simulink model "ex3_2"  (Simulink 7.4)
settings: Solver=FixedStepDiscrete  SolverMode=SingleTasking  StartTime=0.0  StopTime=inf  FixedStep=0.005  RelTol=1e-3
libraries: dspsigops x20, dsparch4 x1
settings Model: Creator=fwornle  LastModifiedBy=fw  SimulationMode=external
settings ConfigSet: Description=rtmc9s12target_R2009b
settings DataIOCC: SignalLoggingName=sigsOut
settings OptimizationCC: InitFltsAndDblsToZero=on  OptimizeModelRefInitCode=on  LifeSpan=1
settings DebuggingCC: SaveWithParameterizedLinksMsg=none  SignalResolutionControl=TryResolveAllWithWarning  SolverPrmCheckMsg=none  MultiTaskDSMMsg=warning  MultiTaskCondExecSysMsg=none  StrictBusMsg=None
settings HardwareCC: ProdBitPerInt=16  ProdEndianess=BigEndian  ProdWordSize=16  ProdHWDeviceType=Motorola HC12
settings RTWCC: SystemTargetFile=mc9s12.tlc  GenerateMakefile=off  TemplateMakefile=mc9s12.tmf  ProcessScript=mc9s12_make_rtw_hook  IncludeERTFirstTime=on
settings STFCustomTargetCC: TargetFcnLib=ansi_tfl_tmw.mat  ModelReferenceCompliant=off  IncludeMdlTerminateFcn=off  ERTCustomFileBanners=on  SupportNonInlinedSFcns=off  CPPClassGenCompliant=on  SystemTargetFile=mc9s12.tlc
settings ERTTargetCC: TargetFcnLib=ansi_tfl_tmw.mat  MultiwordLength=2048  ModelReferenceCompliant=off  ParMdlRefBuildCompliant=off  CompOptLevelCompliant=off  IncludeMdlTerminateFcn=off  CombineOutputUpdateFcns=off  ERTFirstTimeCompliant=off  SupportContinuousTime=on  ModelStepFunctionPrototypeControlCompliant=off  ExtMode=on  ExtModeMexFile=ext_serial_mc9s12_comm  ExtModeMexArgs=1,2,115200  InlinedParameterPlacement=NonHierarchical  ERTCustomFileTemplate=mc9s12_file_process.tlc  GRTInterface=on  ConvertIfToSwitch=off
settings CustomProperty: DataType=RTWOptions_EnumType_C__Users_fw__SVN_rtmc9s12-target_trunk_rtmc9s12_CW_R2009b_bin_mc9s12_1mc9s12_TargetBoard  Value=Dragon12Plus
settings EnumStrPairs: String=Dragon12

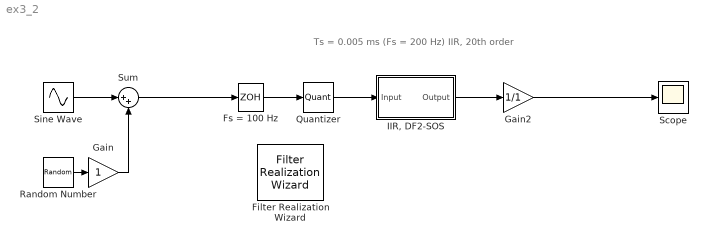
== system ex3_2 ==
  note: Ts = 0.005 ms
      | (Fs = 200 Hz)
      | IIR, 20th order
  Filter Realization Wizard : dsparch4/Filter Realization Wizard  SystemSampleTime=-1
  Fs = 100 Hz : ZeroOrderHold  SampleTime=0.01
  Gain : Gain  ParameterDataType=sfix(16)  ParameterScaling=2^0  OutDataType=sfix(16)  OutScaling=2^0  SaturateOnIntegerOverflow=on  OutDataTypeStr=Inherit: Same as input  ParamDataTypeStr=Inherit: Same as input
  Gain2 : Gain  Gain=1/1  ParameterDataType=sfix(16)  ParameterScaling=2^0  OutDataType=sfix(16)  OutScaling=2^0  SaturateOnIntegerOverflow=on  OutDataTypeStr=Inherit: Same as input  ParamDataTypeStr=Inherit: Same as input
  "IIR, DF2-SOS" : Subsystem  Tag=FilterWizardSubSystem
  Quantizer : Quantizer  QuantizationInterval=2/(2^6-1)  LinearizeAsGain=off
  Random Number : RandomNumber  Variance=1e-6  SampleTime=0
  Scope : Scope
      settings: TimeRange=1  YMin=-1.5  YMax=1.5  SaveName=y1
  Sine Wave : Sin  Amplitude=1  Bias=0  Frequency=2*pi*20  Phase=0  Samples=10  SampleTime=0  Offset=0
  Sum : Sum  Inputs=|++  OutDataType=sfix(16)  OutScaling=2^0  SaturateOnIntegerOverflow=on
  wires:
  Random Number/1 -> Gain/1
  Gain/1 -> Sum/2
  Fs = 100 Hz/1 -> Quantizer/1
  Sine Wave/1 -> Sum/1
  "IIR, DF2-SOS"/1(Output) -> Gain2/1
  Sum/1 -> Fs = 100 Hz/1
  Quantizer/1 -> "IIR, DF2-SOS"/1(Input)
  Gain2/1 -> Scope/1

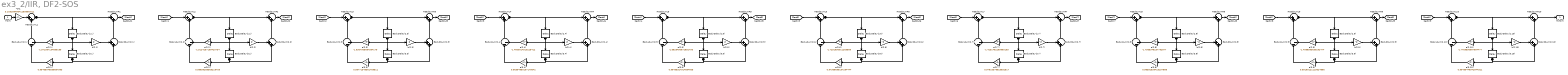
== system ex3_2/IIR, DF2-SOS ==
  Input : Inport  OutDataType=sfix(16)  OutScaling=2^0
  BodyDelay(2,1) : dspsigops/Delay  dly_unit=Samples  delay=1  ic_detail=off  dif_ic_for_ch=off  dif_ic_for_dly=off  ic=0  reset_popup=None
  BodyDelay(2,10) : dspsigops/Delay  dly_unit=Samples  delay=1  ic_detail=off  dif_ic_for_ch=off  dif_ic_for_dly=off  ic=0  reset_popup=None
  BodyDelay(2,2) : dspsigops/Delay  dly_unit=Samples  delay=1  ic_detail=off  dif_ic_for_ch=off  dif_ic_for_dly=off  ic=0  reset_popup=None
  BodyDelay(2,3) : dspsigops/Delay  dly_unit=Samples  delay=1  ic_detail=off  dif_ic_for_ch=off  dif_ic_for_dly=off  ic=0  reset_popup=None
  BodyDelay(2,4) : dspsigops/Delay  dly_unit=Samples  delay=1  ic_detail=off  dif_ic_for_ch=off  dif_ic_for_dly=off  ic=0  reset_popup=None
  BodyDelay(2,5) : dspsigops/Delay  dly_unit=Samples  delay=1  ic_detail=off  dif_ic_for_ch=off  dif_ic_for_dly=off  ic=0  reset_popup=None
  BodyDelay(2,6) : dspsigops/Delay  dly_unit=Samples  delay=1  ic_detail=off  dif_ic_for_ch=off  dif_ic_for_dly=off  ic=0  reset_popup=None
  BodyDelay(2,7) : dspsigops/Delay  dly_unit=Samples  delay=1  ic_detail=off  dif_ic_for_ch=off  dif_ic_for_dly=off  ic=0  reset_popup=None
  BodyDelay(2,8) : dspsigops/Delay  dly_unit=Samples  delay=1  ic_detail=off  dif_ic_for_ch=off  dif_ic_for_dly=off  ic=0  reset_popup=None
  BodyDelay(2,9) : dspsigops/Delay  dly_unit=Samples  delay=1  ic_detail=off  dif_ic_for_ch=off  dif_ic_for_dly=off  ic=0  reset_popup=None
  BodyDelay(3,1) : dspsigops/Delay  dly_unit=Samples  delay=1  ic_detail=off  dif_ic_for_ch=off  dif_ic_for_dly=off  ic=0  reset_popup=None
  BodyDelay(3,10) : dspsigops/Delay  dly_unit=Samples  delay=1  ic_detail=off  dif_ic_for_ch=off  dif_ic_for_dly=off  ic=0  reset_popup=None
  BodyDelay(3,2) : dspsigops/Delay  dly_unit=Samples  delay=1  ic_detail=off  dif_ic_for_ch=off  dif_ic_for_dly=off  ic=0  reset_popup=None
  BodyDelay(3,3) : dspsigops/Delay  dly_unit=Samples  delay=1  ic_detail=off  dif_ic_for_ch=off  dif_ic_for_dly=off  ic=0  reset_popup=None
  BodyDelay(3,4) : dspsigops/Delay  dly_unit=Samples  delay=1  ic_detail=off  dif_ic_for_ch=off  dif_ic_for_dly=off  ic=0  reset_popup=None
  BodyDelay(3,5) : dspsigops/Delay  dly_unit=Samples  delay=1  ic_detail=off  dif_ic_for_ch=off  dif_ic_for_dly=off  ic=0  reset_popup=None
  BodyDelay(3,6) : dspsigops/Delay  dly_unit=Samples  delay=1  ic_detail=off  dif_ic_for_ch=off  dif_ic_for_dly=off  ic=0  reset_popup=None
  BodyDelay(3,7) : dspsigops/Delay  dly_unit=Samples  delay=1  ic_detail=off  dif_ic_for_ch=off  dif_ic_for_dly=off  ic=0  reset_popup=None
  BodyDelay(3,8) : dspsigops/Delay  dly_unit=Samples  delay=1  ic_detail=off  dif_ic_for_ch=off  dif_ic_for_dly=off  ic=0  reset_popup=None
  BodyDelay(3,9) : dspsigops/Delay  dly_unit=Samples  delay=1  ic_detail=off  dif_ic_for_ch=off  dif_ic_for_dly=off  ic=0  reset_popup=None
  BodyLSum(2,1) : Sum  Inputs=|--  OutDataType=sfix(16)  OutScaling=2^0  SaturateOnIntegerOverflow=on  InputSameDT=on  OutDataTypeStr=Inherit: Same as first input
  BodyLSum(2,10) : Sum  Inputs=|--  OutDataType=sfix(16)  OutScaling=2^0  SaturateOnIntegerOverflow=on  InputSameDT=on  OutDataTypeStr=Inherit: Same as first input
  BodyLSum(2,2) : Sum  Inputs=|--  OutDataType=sfix(16)  OutScaling=2^0  SaturateOnIntegerOverflow=on  InputSameDT=on  OutDataTypeStr=Inherit: Same as first input
  BodyLSum(2,3) : Sum  Inputs=|--  OutDataType=sfix(16)  OutScaling=2^0  SaturateOnIntegerOverflow=on  InputSameDT=on  OutDataTypeStr=Inherit: Same as first input
  BodyLSum(2,4) : Sum  Inputs=|--  OutDataType=sfix(16)  OutScaling=2^0  SaturateOnIntegerOverflow=on  InputSameDT=on  OutDataTypeStr=Inherit: Same as first input
  BodyLSum(2,5) : Sum  Inputs=|--  OutDataType=sfix(16)  OutScaling=2^0  SaturateOnIntegerOverflow=on  InputSameDT=on  OutDataTypeStr=Inherit: Same as first input
  BodyLSum(2,6) : Sum  Inputs=|--  OutDataType=sfix(16)  OutScaling=2^0  SaturateOnIntegerOverflow=on  InputSameDT=on  OutDataTypeStr=Inherit: Same as first input
  BodyLSum(2,7) : Sum  Inputs=|--  OutDataType=sfix(16)  OutScaling=2^0  SaturateOnIntegerOverflow=on  InputSameDT=on  OutDataTypeStr=Inherit: Same as first input
  BodyLSum(2,8) : Sum  Inputs=|--  OutDataType=sfix(16)  OutScaling=2^0  SaturateOnIntegerOverflow=on  InputSameDT=on  OutDataTypeStr=Inherit: Same as first input
  BodyLSum(2,9) : Sum  Inputs=|--  OutDataType=sfix(16)  OutScaling=2^0  SaturateOnIntegerOverflow=on  InputSameDT=on  OutDataTypeStr=Inherit: Same as first input
  BodyRSum(2,1) : Sum  Inputs=++|  OutDataType=sfix(16)  OutScaling=2^0  SaturateOnIntegerOverflow=on  InputSameDT=on  OutDataTypeStr=Inherit: Same as first input
  BodyRSum(2,10) : Sum  Inputs=++|  OutDataType=sfix(16)  OutScaling=2^0  SaturateOnIntegerOverflow=on  InputSameDT=on  OutDataTypeStr=Inherit: Same as first input
  BodyRSum(2,2) : Sum  Inputs=++|  OutDataType=sfix(16)  OutScaling=2^0  SaturateOnIntegerOverflow=on  InputSameDT=on  OutDataTypeStr=Inherit: Same as first input
  BodyRSum(2,3) : Sum  Inputs=++|  OutDataType=sfix(16)  OutScaling=2^0  SaturateOnIntegerOverflow=on  InputSameDT=on  OutDataTypeStr=Inherit: Same as first input
  BodyRSum(2,4) : Sum  Inputs=++|  OutDataType=sfix(16)  OutScaling=2^0  SaturateOnIntegerOverflow=on  InputSameDT=on  OutDataTypeStr=Inherit: Same as first input
  BodyRSum(2,5) : Sum  Inputs=++|  OutDataType=sfix(16)  OutScaling=2^0  SaturateOnIntegerOverflow=on  InputSameDT=on  OutDataTypeStr=Inherit: Same as first input
  BodyRSum(2,6) : Sum  Inputs=++|  OutDataType=sfix(16)  OutScaling=2^0  SaturateOnIntegerOverflow=on  InputSameDT=on  OutDataTypeStr=Inherit: Same as first input
  BodyRSum(2,7) : Sum  Inputs=++|  OutDataType=sfix(16)  OutScaling=2^0  SaturateOnIntegerOverflow=on  InputSameDT=on  OutDataTypeStr=Inherit: Same as first input
  BodyRSum(2,8) : Sum  Inputs=++|  OutDataType=sfix(16)  OutScaling=2^0  SaturateOnIntegerOverflow=on  InputSameDT=on  OutDataTypeStr=Inherit: Same as first input
  BodyRSum(2,9) : Sum  Inputs=++|  OutDataType=sfix(16)  OutScaling=2^0  SaturateOnIntegerOverflow=on  InputSameDT=on  OutDataTypeStr=Inherit: Same as first input
  HeadSumL{1..10} (10 alike) : Sum  Inputs=|++  OutDataType=sfix(16)  OutScaling=2^0  SaturateOnIntegerOverflow=on  InputSameDT=on  OutDataTypeStr=Inherit: Same as first input
  HeadSumR{1..10} (10 alike) : Sum  Inputs=|++  OutDataType=sfix(16)  OutScaling=2^0  SaturateOnIntegerOverflow=on  InputSameDT=on  OutDataTypeStr=Inherit: Same as first input
  a(2,1) : Gain  Gain=-1.571957134859189  ParameterDataType=sfix(16)  ParameterScaling=2^0  OutDataType=sfix(16)  OutScaling=2^0  SaturateOnIntegerOverflow=on  OutDataTypeStr=Inherit: Same as input  ParamDataTypeStr=Inherit: Same as input
  a(2,10) : Gain  Gain=-1.7769550987684477  ParameterDataType=sfix(16)  ParameterScaling=2^0  OutDataType=sfix(16)  OutScaling=2^0  SaturateOnIntegerOverflow=on  OutDataTypeStr=Inherit: Same as input  ParamDataTypeStr=Inherit: Same as input
  a(2,2) : Gain  Gain=-1.5124257199420734  ParameterDataType=sfix(16)  ParameterScaling=2^0  OutDataType=sfix(16)  OutScaling=2^0  SaturateOnIntegerOverflow=on  OutDataTypeStr=Inherit: Same as input  ParamDataTypeStr=Inherit: Same as input
  a(2,3) : Gain  Gain=-1.6307005687554179  ParameterDataType=sfix(16)  ParameterScaling=2^0  OutDataType=sfix(16)  OutScaling=2^0  SaturateOnIntegerOverflow=on  OutDataTypeStr=Inherit: Same as input  ParamDataTypeStr=Inherit: Same as input
  a(2,4) : Gain  Gain=-1.4600014510225412  ParameterDataType=sfix(16)  ParameterScaling=2^0  OutDataType=sfix(16)  OutScaling=2^0  SaturateOnIntegerOverflow=on  OutDataTypeStr=Inherit: Same as input  ParamDataTypeStr=Inherit: Same as input
  a(2,5) : Gain  Gain=-1.6828450672852706  ParameterDataType=sfix(16)  ParameterScaling=2^0  OutDataType=sfix(16)  OutScaling=2^0  SaturateOnIntegerOverflow=on  OutDataTypeStr=Inherit: Same as input  ParamDataTypeStr=Inherit: Same as input
  a(2,6) : Gain  Gain=-1.7251650011265589  ParameterDataType=sfix(16)  ParameterScaling=2^0  OutDataType=sfix(16)  OutScaling=2^0  SaturateOnIntegerOverflow=on  OutDataTypeStr=Inherit: Same as input  ParamDataTypeStr=Inherit: Same as input
  a(2,7) : Gain  Gain=-1.4231462269960193  ParameterDataType=sfix(16)  ParameterScaling=2^0  OutDataType=sfix(16)  OutScaling=2^0  SaturateOnIntegerOverflow=on  OutDataTypeStr=Inherit: Same as input  ParamDataTypeStr=Inherit: Same as input
  a(2,8) : Gain  Gain=-1.7565348237792877  ParameterDataType=sfix(16)  ParameterScaling=2^0  OutDataType=sfix(16)  OutScaling=2^0  SaturateOnIntegerOverflow=on  OutDataTypeStr=Inherit: Same as input  ParamDataTypeStr=Inherit: Same as input
  a(2,9) : Gain  Gain=-1.4088593630292474  ParameterDataType=sfix(16)  ParameterScaling=2^0  OutDataType=sfix(16)  OutScaling=2^0  SaturateOnIntegerOverflow=on  OutDataTypeStr=Inherit: Same as input  ParamDataTypeStr=Inherit: Same as input
  a(3,1) : Gain  Gain=0.95465049539857993  ParameterDataType=sfix(16)  ParameterScaling=2^0  OutDataType=sfix(16)  OutScaling=2^0  SaturateOnIntegerOverflow=on  OutDataTypeStr=Inherit: Same as input  ParamDataTypeStr=Inherit: Same as input
  a(3,10) : Gain  Gain=0.99459446942844321  ParameterDataType=sfix(16)  ParameterScaling=2^0  OutDataType=sfix(16)  OutScaling=2^0  SaturateOnIntegerOverflow=on  OutDataTypeStr=Inherit: Same as input  ParamDataTypeStr=Inherit: Same as input
  a(3,2) : Gain  Gain=0.95659285365218705  ParameterDataType=sfix(16)  ParameterScaling=2^0  OutDataType=sfix(16)  OutScaling=2^0  SaturateOnIntegerOverflow=on  OutDataTypeStr=Inherit: Same as input  ParamDataTypeStr=Inherit: Same as input
  a(3,3) : Gain  Gain=0.95771345361769511  ParameterDataType=sfix(16)  ParameterScaling=2^0  OutDataType=sfix(16)  OutScaling=2^0  SaturateOnIntegerOverflow=on  OutDataTypeStr=Inherit: Same as input  ParamDataTypeStr=Inherit: Same as input
  a(3,4) : Gain  Gain=0.96394950197178042  ParameterDataType=sfix(16)  ParameterScaling=2^0  OutDataType=sfix(16)  OutScaling=2^0  SaturateOnIntegerOverflow=on  OutDataTypeStr=Inherit: Same as input  ParamDataTypeStr=Inherit: Same as input
  a(3,5) : Gain  Gain=0.96455327914854605  ParameterDataType=sfix(16)  ParameterScaling=2^0  OutDataType=sfix(16)  OutScaling=2^0  SaturateOnIntegerOverflow=on  OutDataTypeStr=Inherit: Same as input  ParamDataTypeStr=Inherit: Same as input
  a(3,6) : Gain  Gain=0.97368699157284444  ParameterDataType=sfix(16)  ParameterScaling=2^0  OutDataType=sfix(16)  OutScaling=2^0  SaturateOnIntegerOverflow=on  OutDataTypeStr=Inherit: Same as input  ParamDataTypeStr=Inherit: Same as input
  a(3,7) : Gain  Gain=0.97610378923932517  ParameterDataType=sfix(16)  ParameterScaling=2^0  OutDataType=sfix(16)  OutScaling=2^0  SaturateOnIntegerOverflow=on  OutDataTypeStr=Inherit: Same as input  ParamDataTypeStr=Inherit: Same as input
  a(3,8) : Gain  Gain=0.98392539423157888  ParameterDataType=sfix(16)  ParameterScaling=2^0  OutDataType=sfix(16)  OutScaling=2^0  SaturateOnIntegerOverflow=on  OutDataTypeStr=Inherit: Same as input  ParamDataTypeStr=Inherit: Same as input
  a(3,9) : Gain  Gain=0.99160121115624866  ParameterDataType=sfix(16)  ParameterScaling=2^0  OutDataType=sfix(16)  OutScaling=2^0  SaturateOnIntegerOverflow=on  OutDataTypeStr=Inherit: Same as input  ParamDataTypeStr=Inherit: Same as input
  b(2,1) : Gain  Gain=2  ParameterDataType=sfix(16)  ParameterScaling=2^0  OutDataType=sfix(16)  OutScaling=2^0  SaturateOnIntegerOverflow=on  OutDataTypeStr=Inherit: Same as input  ParamDataTypeStr=Inherit: Same as input
  b(2,10) : Gain  Gain=-2  ParameterDataType=sfix(16)  ParameterScaling=2^0  OutDataType=sfix(16)  OutScaling=2^0  SaturateOnIntegerOverflow=on  OutDataTypeStr=Inherit: Same as input  ParamDataTypeStr=Inherit: Same as input
  b(2,2) : Gain  Gain=2  ParameterDataType=sfix(16)  ParameterScaling=2^0  OutDataType=sfix(16)  OutScaling=2^0  SaturateOnIntegerOverflow=on  OutDataTypeStr=Inherit: Same as input  ParamDataTypeStr=Inherit: Same as input
  b(2,3) : Gain  Gain=2  ParameterDataType=sfix(16)  ParameterScaling=2^0  OutDataType=sfix(16)  OutScaling=2^0  SaturateOnIntegerOverflow=on  OutDataTypeStr=Inherit: Same as input  ParamDataTypeStr=Inherit: Same as input
  b(2,4) : Gain  Gain=2  ParameterDataType=sfix(16)  ParameterScaling=2^0  OutDataType=sfix(16)  OutScaling=2^0  SaturateOnIntegerOverflow=on  OutDataTypeStr=Inherit: Same as input  ParamDataTypeStr=Inherit: Same as input
  b(2,5) : Gain  Gain=2  ParameterDataType=sfix(16)  ParameterScaling=2^0  OutDataType=sfix(16)  OutScaling=2^0  SaturateOnIntegerOverflow=on  OutDataTypeStr=Inherit: Same as input  ParamDataTypeStr=Inherit: Same as input
  b(2,6) : Gain  Gain=-2  ParameterDataType=sfix(16)  ParameterScaling=2^0  OutDataType=sfix(16)  OutScaling=2^0  SaturateOnIntegerOverflow=on  OutDataTypeStr=Inherit: Same as input  ParamDataTypeStr=Inherit: Same as input
  b(2,7) : Gain  Gain=-2  ParameterDataType=sfix(16)  ParameterScaling=2^0  OutDataType=sfix(16)  OutScaling=2^0  SaturateOnIntegerOverflow=on  OutDataTypeStr=Inherit: Same as input  ParamDataTypeStr=Inherit: Same as input
  b(2,8) : Gain  Gain=-2  ParameterDataType=sfix(16)  ParameterScaling=2^0  OutDataType=sfix(16)  OutScaling=2^0  SaturateOnIntegerOverflow=on  OutDataTypeStr=Inherit: Same as input  ParamDataTypeStr=Inherit: Same as input
  b(2,9) : Gain  Gain=-2  ParameterDataType=sfix(16)  ParameterScaling=2^0  OutDataType=sfix(16)  OutScaling=2^0  SaturateOnIntegerOverflow=on  OutDataTypeStr=Inherit: Same as input  ParamDataTypeStr=Inherit: Same as input
  s(1) : Gain  Gain=3.1031894864125959e-011  ParameterDataType=sfix(16)  ParameterScaling=2^0  OutDataType=sfix(16)  OutScaling=2^0  SaturateOnIntegerOverflow=on  OutDataTypeStr=Inherit: Same as input  ParamDataTypeStr=Inherit: Same as input
  Output : Outport  OutDataType=sfix(16)  OutScaling=2^0
  wires:
  Input/1 -> s(1)/1
  s(1)/1 -> HeadSumL1/1
  HeadSumL1/1 -> BodyDelay(2,1)/1, HeadSumR1/1
  HeadSumR1/1 -> [Sect1]
  BodyDelay(2,1)/1 -> a(2,1)/1, b(2,1)/1, BodyDelay(3,1)/1
  a(2,1)/1 -> BodyLSum(2,1)/2
  b(2,1)/1 -> BodyRSum(2,1)/1
  BodyLSum(2,1)/1 -> HeadSumL1/2
  BodyRSum(2,1)/1 -> HeadSumR1/2
  BodyDelay(3,1)/1 -> a(3,1)/1, BodyRSum(2,1)/2
  a(3,1)/1 -> BodyLSum(2,1)/1
  [Sect1] -> HeadSumL2/1
  HeadSumL2/1 -> BodyDelay(2,2)/1, HeadSumR2/1
  HeadSumR2/1 -> [Sect2]
  BodyDelay(2,2)/1 -> a(2,2)/1, b(2,2)/1, BodyDelay(3,2)/1
  a(2,2)/1 -> BodyLSum(2,2)/2
  b(2,2)/1 -> BodyRSum(2,2)/1
  BodyLSum(2,2)/1 -> HeadSumL2/2
  BodyRSum(2,2)/1 -> HeadSumR2/2
  BodyDelay(3,2)/1 -> a(3,2)/1, BodyRSum(2,2)/2
  a(3,2)/1 -> BodyLSum(2,2)/1
  [Sect2] -> HeadSumL3/1
  HeadSumL3/1 -> BodyDelay(2,3)/1, HeadSumR3/1
  HeadSumR3/1 -> [Sect3]
  BodyDelay(2,3)/1 -> a(2,3)/1, b(2,3)/1, BodyDelay(3,3)/1
  a(2,3)/1 -> BodyLSum(2,3)/2
  b(2,3)/1 -> BodyRSum(2,3)/1
  BodyLSum(2,3)/1 -> HeadSumL3/2
  BodyRSum(2,3)/1 -> HeadSumR3/2
  BodyDelay(3,3)/1 -> a(3,3)/1, BodyRSum(2,3)/2
  a(3,3)/1 -> BodyLSum(2,3)/1
  [Sect3] -> HeadSumL4/1
  HeadSumL4/1 -> BodyDelay(2,4)/1, HeadSumR4/1
  HeadSumR4/1 -> [Sect4]
  BodyDelay(2,4)/1 -> a(2,4)/1, b(2,4)/1, BodyDelay(3,4)/1
  a(2,4)/1 -> BodyLSum(2,4)/2
  b(2,4)/1 -> BodyRSum(2,4)/1
  BodyLSum(2,4)/1 -> HeadSumL4/2
  BodyRSum(2,4)/1 -> HeadSumR4/2
  BodyDelay(3,4)/1 -> a(3,4)/1, BodyRSum(2,4)/2
  a(3,4)/1 -> BodyLSum(2,4)/1
  [Sect4] -> HeadSumL5/1
  HeadSumL5/1 -> BodyDelay(2,5)/1, HeadSumR5/1
  HeadSumR5/1 -> [Sect5]
  BodyDelay(2,5)/1 -> a(2,5)/1, b(2,5)/1, BodyDelay(3,5)/1
  a(2,5)/1 -> BodyLSum(2,5)/2
  b(2,5)/1 -> BodyRSum(2,5)/1
  BodyLSum(2,5)/1 -> HeadSumL5/2
  BodyRSum(2,5)/1 -> HeadSumR5/2
  BodyDelay(3,5)/1 -> a(3,5)/1, BodyRSum(2,5)/2
  a(3,5)/1 -> BodyLSum(2,5)/1
  [Sect5] -> HeadSumL6/1
  HeadSumL6/1 -> BodyDelay(2,6)/1, HeadSumR6/1
  HeadSumR6/1 -> [Sect6]
  BodyDelay(2,6)/1 -> a(2,6)/1, b(2,6)/1, BodyDelay(3,6)/1
  a(2,6)/1 -> BodyLSum(2,6)/2
  b(2,6)/1 -> BodyRSum(2,6)/1
  BodyLSum(2,6)/1 -> HeadSumL6/2
  BodyRSum(2,6)/1 -> HeadSumR6/2
  BodyDelay(3,6)/1 -> a(3,6)/1, BodyRSum(2,6)/2
  a(3,6)/1 -> BodyLSum(2,6)/1
  [Sect6] -> HeadSumL7/1
  HeadSumL7/1 -> BodyDelay(2,7)/1, HeadSumR7/1
  HeadSumR7/1 -> [Sect7]
  BodyDelay(2,7)/1 -> a(2,7)/1, b(2,7)/1, BodyDelay(3,7)/1
  a(2,7)/1 -> BodyLSum(2,7)/2
  b(2,7)/1 -> BodyRSum(2,7)/1
  BodyLSum(2,7)/1 -> HeadSumL7/2
  BodyRSum(2,7)/1 -> HeadSumR7/2
  BodyDelay(3,7)/1 -> a(3,7)/1, BodyRSum(2,7)/2
  a(3,7)/1 -> BodyLSum(2,7)/1
  [Sect7] -> HeadSumL8/1
  HeadSumL8/1 -> BodyDelay(2,8)/1, HeadSumR8/1
  HeadSumR8/1 -> [Sect8]
  BodyDelay(2,8)/1 -> a(2,8)/1, b(2,8)/1, BodyDelay(3,8)/1
  a(2,8)/1 -> BodyLSum(2,8)/2
  b(2,8)/1 -> BodyRSum(2,8)/1
  BodyLSum(2,8)/1 -> HeadSumL8/2
  BodyRSum(2,8)/1 -> HeadSumR8/2
  BodyDelay(3,8)/1 -> a(3,8)/1, BodyRSum(2,8)/2
  a(3,8)/1 -> BodyLSum(2,8)/1
  [Sect8] -> HeadSumL9/1
  HeadSumL9/1 -> BodyDelay(2,9)/1, HeadSumR9/1
  HeadSumR9/1 -> [Sect9]
  BodyDelay(2,9)/1 -> a(2,9)/1, b(2,9)/1, BodyDelay(3,9)/1
  a(2,9)/1 -> BodyLSum(2,9)/2
  b(2,9)/1 -> BodyRSum(2,9)/1
  BodyLSum(2,9)/1 -> HeadSumL9/2
  BodyRSum(2,9)/1 -> HeadSumR9/2
  BodyDelay(3,9)/1 -> a(3,9)/1, BodyRSum(2,9)/2
  a(3,9)/1 -> BodyLSum(2,9)/1
  [Sect9] -> HeadSumL10/1
  HeadSumL10/1 -> BodyDelay(2,10)/1, HeadSumR10/1
  HeadSumR10/1 -> Output/1
  BodyDelay(2,10)/1 -> a(2,10)/1, b(2,10)/1, BodyDelay(3,10)/1
  a(2,10)/1 -> BodyLSum(2,10)/2
  b(2,10)/1 -> BodyRSum(2,10)/1
  BodyLSum(2,10)/1 -> HeadSumL10/2
  BodyRSum(2,10)/1 -> HeadSumR10/2
  BodyDelay(3,10)/1 -> a(3,10)/1, BodyRSum(2,10)/2
  a(3,10)/1 -> BodyLSum(2,10)/1
